simulink model "f1"  (R2014a)
settings: Solver=ode45  StartTime=0.0  StopTime=5  RelTol=1e-3
settings Model: Creator=root  LastModifiedBy=root

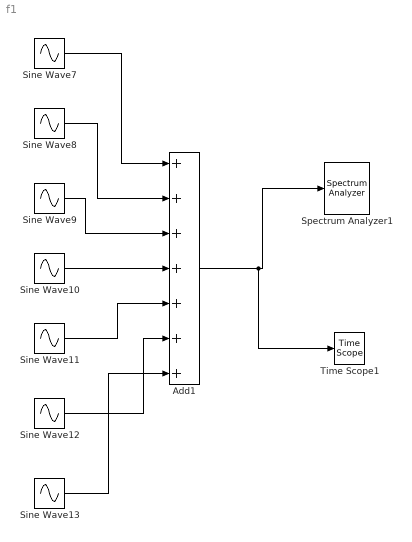
== system f1 ==
  Add1 : Sum  Inputs=+++++++
  Sine Wave10 : Sin  Amplitude=0  Frequency=8*pi  SampleTime=0.001
  Sine Wave11 : Sin  Amplitude=8/(pi*pi)  Frequency=10*pi  SampleTime=0.001
  Sine Wave12 : Sin  Amplitude=0  Frequency=12*pi  SampleTime=0.001
  Sine Wave13 : Sin  Amplitude=-8/(pi*pi)  Frequency=14*pi  SampleTime=0.001
  Sine Wave7 : Sin  Amplitude=8/(pi*pi)  Frequency=2*pi  SampleTime=0.001
  Sine Wave8 : Sin  Amplitude=0  Frequency=4*pi  SampleTime=0.001
  Sine Wave9 : Sin  Amplitude=-8/(pi*pi)  Frequency=6*pi  SampleTime=0.001
  Spectrum Analyzer1 : SpectrumAnalyzer
  Time Scope1 : TimeScope  DefaultConfigurationName=spbscopes.TimeScopeBlockCfg
  wires:
  Sine Wave7/1 -> Add1/1
  Sine Wave8/1 -> Add1/2
  Sine Wave9/1 -> Add1/3
  Sine Wave10/1 -> Add1/4
  Sine Wave11/1 -> Add1/5
  Sine Wave12/1 -> Add1/6
  Sine Wave13/1 -> Add1/7
  Add1/1 -> Time Scope1/1, Spectrum Analyzer1/1
